simulink model "uporabne_funkcije"  (R2019b)
settings: Solver=VariableStepAuto  StartTime=0.0  StopTime=10.0  RelTol=1e-3
libraries: simulink x1
settings Model: Creator=student  LastModifiedBy=student

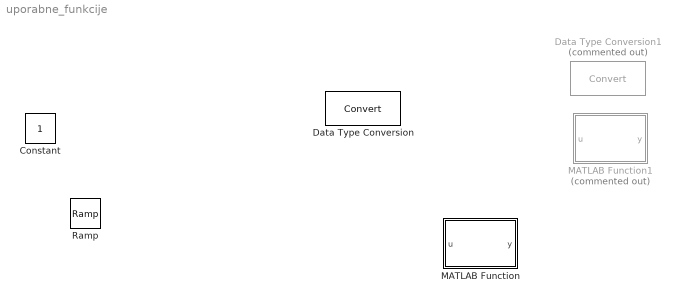
== system uporabne_funkcije ==
  Constant : Constant
  Data Type Conversion : DataTypeConversion
  Data Type Conversion1 : DataTypeConversion  Commented=on
  MATLAB Function : MATLAB Function  TreatAsAtomicUnit=on
  MATLAB Function1 : MATLAB Function  Commented=on  TreatAsAtomicUnit=on
  Ramp : simulink/Sources/Ramp  slope=1  start=0  InitialOutput=0

== matlab function uporabne_funkcije/MATLAB Function1 ==
  data: u input; y output
function y = fcn(u)

y = u;

== matlab function uporabne_funkcije/MATLAB Function ==
  data: u input; y output
function y = fcn(u)

y = u;
